simulink model "gm_bch_encoder_model_fil"  (R2020b)
settings: Solver=FixedStepDiscrete  StartTime=0.0  StopTime=1  RelTol=1e-3
values from neighbouring files (symbols this model uses):
  lfsr_message = [message; false(192, 1)]    [bch_encoder.m]    (also in bch_lfsr_encode_test.m = [message; zeros(n-k, 1)])
libraries: simulink x1, whdlio x1, hdlsllib x1, fillib x1
settings Model: Creator=EFlores  LastModifiedBy=wardo
settings DataIOCC: LimitDataPoints=on  SaveOutput=off  SaveTime=off
settings OptimizationCC: BlockReduction=off  ConditionallyExecuteInputs=off  DefaultParameterBehavior=Inlined  LifeSpan=inf
settings DebuggingCC: AlgebraicLoopMsg=error  InheritedTsInSrcMsg=none  SingleTaskRateTransMsg=error  AllowSymbolicDim=off  StrictBusMsg=ErrorOnBusTreatedAsVector  SFUnexpectedBacktrackingDiag=warning  SFNoUnconditionalDefaultTransitionDiag=warning  SFExecutionAtInitializationDiag=none  ArithmeticOperatorsInVariantConditions=warning
settings HardwareCC: ProdBitPerPointer=32  ProdBitPerSizeT=32  ProdBitPerPtrDiffT=32  ProdLargestAtomicFloat=None  ProdIntDivRoundTo=Undefined  ProdEndianess=Unspecified  ProdWordSize=32  ProdHWDeviceType=ASIC/FPGA->ASIC/FPGA  ProdEqTarget=off
settings SFSimCC: SimUseLocalCustomCode=off  CustomCodeUndefinedFunction=UseInterfaceOnly
settings RTWCC: RTWUseLocalCustomCode=off
settings CodeAppCC: StateflowObjectComments=on
settings GRTTargetCC: TargetLangStandard=C89/C90 (ANSI)
settings ConfigComp: CovScope=ReferencedModels  CovMetricSettings=dw  CovSaveCumulativeToWorkspaceVar=on  CovSaveSingleToWorkspaceVar=on  CovExternalEMLEnable=off  CovSFcnEnable=off

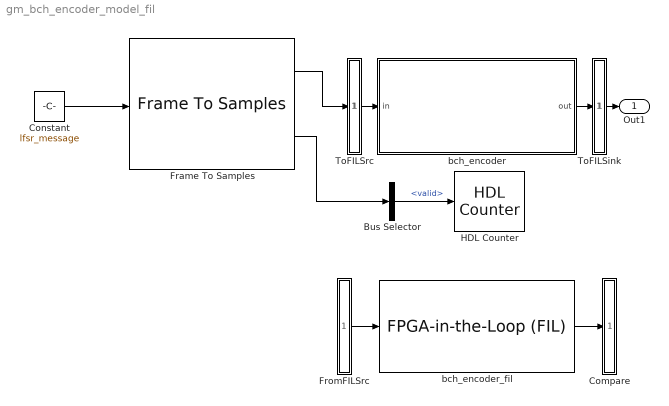
== system gm_bch_encoder_model_fil ==
  Bus Selector : BusSelector  OutputSignals=valid
  Compare : Subsystem
      mask Display: disp('')
  Constant : Constant  Value=lfsr_message  OutDataTypeStr=fixdt(0,1,0)  SampleTime=1
  Frame To Samples : whdlio/Frame To Samples  InterSampleIdleCycles=0  InterFrameIdleCycles=0  OutputSize=1  InterleaveSamples=off
      settings: SourceProductBaseCode=LH
  FromFILSrc : Subsystem
      mask Display: disp('')
  HDL Counter : hdlsllib/Sources/HDL Counter  CountType=Count limited  CountInit=1  CountStep=1  CountMax=48600  CountFromType=Initial value  CountFrom=1  CountResetPort=off  CountLoadPort=off  CountEnbPort=on  CountDirPort=off  CountDataType=Unsigned  CountWordLen=16  CountFracLen=0  CountSampTime=1
  ToFILSink : Subsystem
      mask Display: disp('')
  ToFILSrc : Subsystem
      mask Display: disp('')
  bch_encoder : Subsystem
  bch_encoder_fil : fillib/FPGA-in-the-Loop (FIL)  ForceInterfaceUpdate=0.90579
      settings: SourceProductBaseCode=ES,HD
  Out1 : Outport  VectorParamsAs1DForOutWhenUnconnected=off
  wires:
  Constant/1 -> Frame To Samples/1
  Frame To Samples/2 -> Bus Selector/1
  Bus Selector/1 -> HDL Counter/1  "<valid>"
  ToFILSrc/1(out1) -> bch_encoder/1(in)
  bch_encoder/1(out) -> ToFILSink/1(in1)
  Frame To Samples/1 -> ToFILSrc/1(in1)
  ToFILSink/1(out1) -> Out1/1
  FromFILSrc/1(out1) -> bch_encoder_fil/1
  bch_encoder_fil/1 -> Compare/1(in1)

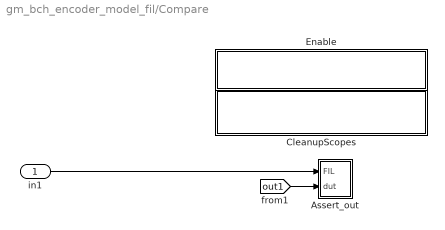
== system gm_bch_encoder_model_fil/Compare ==
  in1 : Inport
  Assert_out : Subsystem
  CleanupScopes : Subsystem
      settings: OpenFcn=|
      | blkName = gcb; %self block
      | idx = regexp(blkName, '/CleanupScopes$', 'once');
      | blkParent = blkName(1:idx-1);
      | blks=find_system(blkParent, 'LookUnderMasks', 'all','blocktype', 'Scope');
      | for itr = 1:length(blks)
      | 	 hScopeCfg = get_param(blks{itr},'ScopeConfiguration');
      | 	 hScopeCfg.Visible = ~ hScopeCfg.Visible;
      | end
      | drawnow;
      mask Display: fprintf(message('hdlcoder:cosim:vnl_dblclick').getString());
  Enable : Subsystem
      settings: OpenFcn=|
      | blkName = gcb;
      | idx = regexp(blkName, '/Enable$', 'once');
      | blkParent = blkName(1:idx-1);
      | blks=find_system(blkParent, 'LookUnderMasks', 'all','blocktype', 'Assertion');
      | e = get_param(blks{1}, 'Enabled');
      | if strcmp(e, 'on'), f= 'off';, else, f = 'on';, end
      | for ii=1:length(blks), set_param(blks{ii}, 'Enabled', f);, end
      | set_param(gcb, 'MaskDisplay',['fprintf(message(''hdlcoder:cosim:vnl_dblclick_assertions'',','''',upper(e),'''',').getString())']);
      mask Display: fprintf(message('hdlcoder:cosim:vnl_dblclick_assertions','OFF').getString());
  wires:
  in1/1 -> Assert_out/1(FIL)
  [out1] -> Assert_out/2(dut)

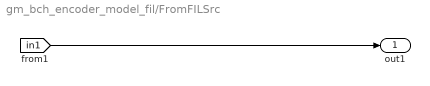
== system gm_bch_encoder_model_fil/FromFILSrc ==
  out1 : Outport
  wires:
  [in1] -> out1/1

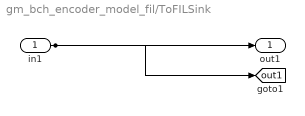
== system gm_bch_encoder_model_fil/ToFILSink ==
  in1 : Inport
  out1 : Outport
  tag scope: out1=global
  wires:
  in1/1 -> out1/1, [out1]

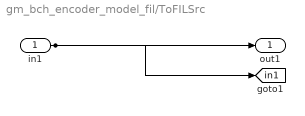
== system gm_bch_encoder_model_fil/ToFILSrc ==
  in1 : Inport
  out1 : Outport
  tag scope: in1=global
  wires:
  in1/1 -> out1/1, [in1]

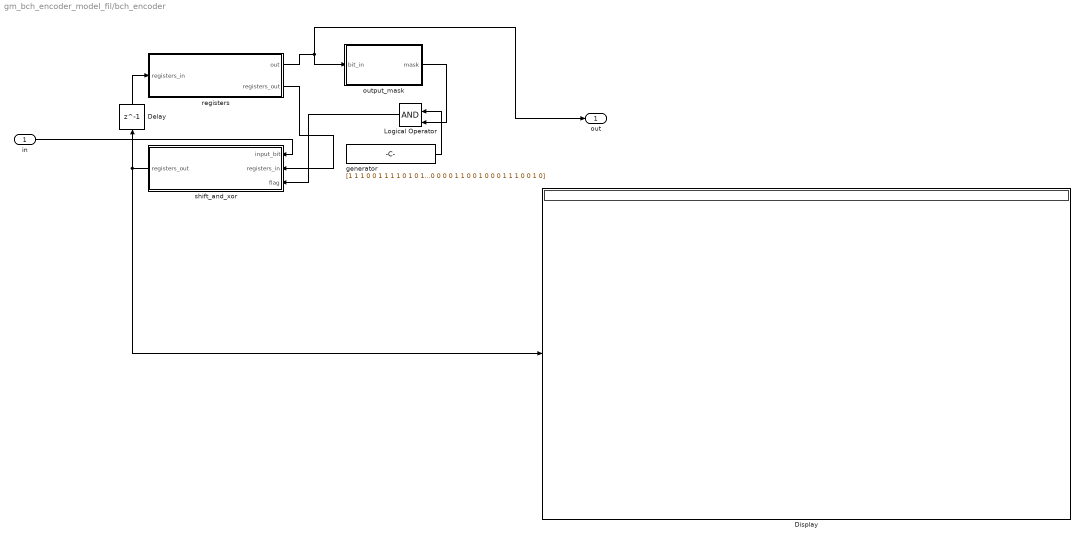
== system gm_bch_encoder_model_fil/bch_encoder ==
  in : Inport
  Delay : Delay  DelayLength=1
  Display : Display
  Logical Operator : Logic  IconShape=distinctive  AllPortsSameDT=off  OutDataTypeStr=fixdt(0, 1, 0)
  generator : Constant  Value=|  OutDataTypeStr=fixdt(0, 1, 0)  SampleTime=-1
      | [1
      | 1
      | 1
      | 0
      | 0
      | 1
      | 1
      | 1
      | 1
      | 0
      | 1
      | 0
      | 1
      | 0
      | 1
      | 0
      | 0
      | 1
      | 0
      | 0
      | 0
      | 0
      | 0
      | 0
      | 0
      | 1
      | 1
      | 0
      | 0
      | 1
      | 1
      | 0
      | 1
      | 1
      | 1
      | 0
      | 1
      | 1
      | 1
      | 1
      | 1
      | 0
      | 1
      | 0
      | 0
      | 0
      | 0
      | 1
      | 1
      | 1
      | 1
      | 0
      | 0
      | 0
      | 1
      | 0
      | 1
      | 1
      | 0
      | 0
      | 0
      | 0
      | 0
      | 0
      | 1
      | 0
      | 0
      | 1
      | 0
      | 0
      | 0
      | 1
      | 0
      | 0
      | 0
      | 1
      | 0
      | 0
      | 0
      | 0
      | 1
      | 0
      | 1
      | 0
      | 1
      | 1
      | 0
      | 0
      | 0
      | 0
      | 1
      | 1
      | 1
      | 0
      | 1
      | 1
      | 0
      | 0
      | 0
      | 1
      | 1
      | 0
      | 1
      | 1
      | 0
      | 0
      | 1
      | 1
      | 0
      | 1
      | 0
      | 0
      | 1
      | 1
      | 1
      | 1
      | 0
      | 0
      | 1
      | 1
      | 0
      | 0
      | 0
      | 0
      | 1
      | 0
      | 1
      | 0
      | 0
      | 0
      | 1
      | 1
      | 1
      | 0
      | 0
      | 0
      | 1
      | 0
      | 0
      | 0
      | 1
      | 0
      | 1
      | 0
      | 0
      | 0
      | 1
      | 1
      | 1
      | 0
      | 1
      | 0
      | 0
      | 0
      | 1
      | 0
      | 0
      | 0
      | 0
      | 1
      | 1
      | 1
      | 0
      | 0
      | 0
      | 0
      | 0
      | 1
      | 0
      | 1
      | 1
      | 1
      | 0
      | 0
      | 0
      | 0
      | 0
      | 1
      | 1
      | 0
      | 0
      | 1
      | 0
      | 0
      | 0
      | 1
      | 1
      | 1
      | 0
      | 0
      | 1
      | 0]
  output_mask : MATLAB Function  TreatAsAtomicUnit=on
  registers : MATLAB Function  TreatAsAtomicUnit=on
  shift_and_xor : MATLAB Function  TreatAsAtomicUnit=on
  out : Outport  VectorParamsAs1DForOutWhenUnconnected=off
  wires:
  registers/1(out) -> out/1, output_mask/1(bit_in)
  output_mask/1(mask) -> Logical Operator/2
  generator/1 -> Logical Operator/1
  Logical Operator/1 -> shift_and_xor/3(flag)
  registers/2(registers_out) -> shift_and_xor/2(registers_in)
  shift_and_xor/1(registers_out) -> Display/1, Delay/1
  in/1 -> shift_and_xor/1(input_bit)
  Delay/1 -> registers/1(registers_in)

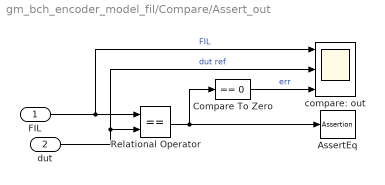
== system gm_bch_encoder_model_fil/Compare/Assert_out ==
  FIL : Inport
  dut : Inport  Port=2
  AssertEq : Assertion  StopWhenAssertionFail=off
  Compare To Zero : simulink/Logic and Bit Operations/Compare To Zero  relop===  OutDataTypeStr=boolean
  Relational Operator : RelationalOperator  Operator===  OutDataTypeStr=boolean  RndMeth=Nearest
  compare: out : Scope  NumInputPorts=3
  wires:
  Compare To Zero/1 -> compare: out/3  "err"
  Relational Operator/1 -> Compare To Zero/1, AssertEq/1
  FIL/1 -> compare: out/1, Relational Operator/1  "FIL"
  dut/1 -> compare: out/2, Relational Operator/2  "dut ref"

== system gm_bch_encoder_model_fil/Compare/CleanupScopes ==

== system gm_bch_encoder_model_fil/Compare/Enable ==

== matlab function gm_bch_encoder_model_fil/bch_encoder/registers ==
  settings: fimath=fimath('RoundingMethod', 'Floor','OverflowAction', 'Wrap','ProductMode', 'FullPrecision', 'SumMode', 'FullPrecision')
  data: registers_in input; out output fixdt(0,1,0) size=1; registers_out output fixdt(0,1,0) size=192
function [out, registers_out] = state_registers(registers_in)
%#codegen

persistent lfsr;
if isempty(lfsr)
    lfsr = fi(zeros(192, 1), 0, 1, 0);
else
    lfsr = registers_in;
end
out = lfsr(192);
registers_out = lfsr;

== matlab function gm_bch_encoder_model_fil/bch_encoder/output_mask ==
  settings: fimath=fimath('RoundingMethod', 'Floor','OverflowAction', 'Wrap','ProductMode', 'FullPrecision', 'SumMode', 'FullPrecision')
  data: bit_in input; mask output
function mask = bitmask(bit_in)
%#codegen

if bit_in
    mask = fi(ones(192, 1), 0, 1, 0);
else
    mask = fi(zeros(192, 1), 0, 1, 0);
end

== matlab function gm_bch_encoder_model_fil/bch_encoder/shift_and_xor ==
  settings: fimath=fimath('RoundingMethod', 'Floor','OverflowAction', 'Wrap','ProductMode', 'FullPrecision', 'SumMode', 'FullPrecision')
  data: input_bit input; registers_out output fixdt(0,1,0); registers_in input; flag input
function registers_out = shift_and_xor(input_bit, registers_in, flag)
%#codegen

buffer = [input_bit; registers_in(1:192-1)];
registers_out = fi(xor(buffer, flag), 0, 1, 0);
